simulink model "SrmUnlineSplineMat3"  (R2013b)
settings: Solver=ode45  StartTime=0.0  StopTime=2  MaxStep=5e-5  RelTol=1e-3
libraries: powerlib x26
settings Model: Creator=Administrator  LastModifiedBy=Think79
settings DataIOCC: SignalLoggingSaveFormat=ModelDataLogs
settings OptimizationCC: ExpressionDepthLimit=2147483647
settings DebuggingCC: FcnCallInpInsideContextMsg=UseLocalSettings  StateNameClashWarn=warning
settings GRTTargetCC: CombineOutputUpdateFcns=off  GRTInterface=on

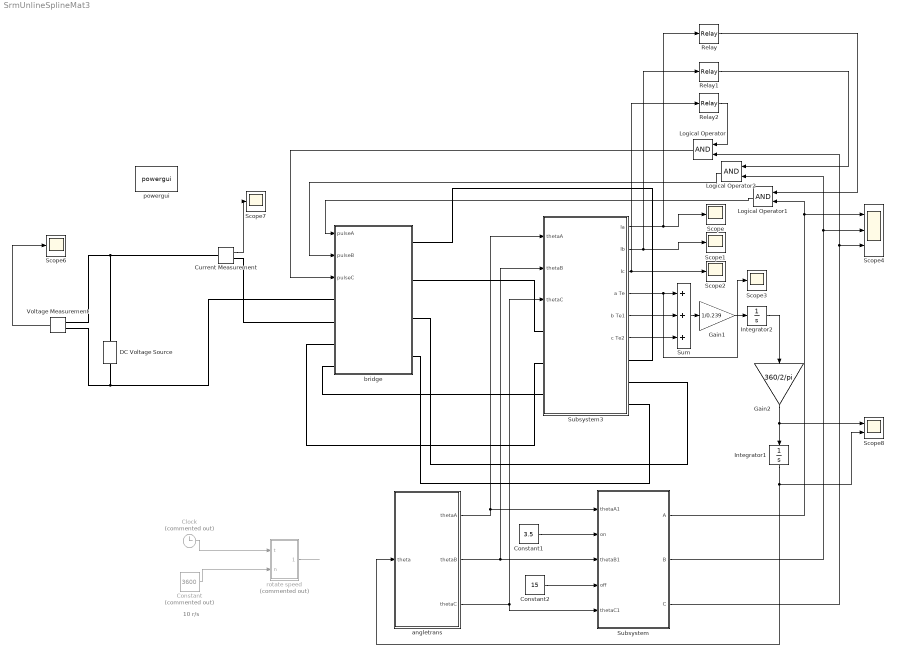
== system SrmUnlineSplineMat3 ==
  note: 10 r/s
  Clock : Clock  Commented=on
  Constant : Constant  Commented=on  Value=3600
  Constant1 : Constant  Value=3.5
  Constant2 : Constant  Value=15
  Current Measurement : powerlib/Measurements/Current Measurement  PhasorSimulation=off  OutputType=Complex  PSBequivalent=0
  DC Voltage Source : powerlib/Electrical Sources/DC Voltage Source  Amplitude=450  Measurements=None
  Gain1 : Gain  Gain=1/0.239
  Gain2 : Gain  Gain=360/2/pi
  Integrator1 : Integrator  InitialCondition=3.5
  Integrator2 : Integrator
  Logical Operator : Logic  AllPortsSameDT=off  OutDataTypeStr=boolean
  Logical Operator1 : Logic  AllPortsSameDT=off  OutDataTypeStr=boolean
  Logical Operator2 : Logic  AllPortsSameDT=off  OutDataTypeStr=boolean
  Relay : Relay  OnSwitchValue=32  OffSwitchValue=28  OnOutputValue=0  OffOutputValue=1
  Relay1 : Relay  OnSwitchValue=32  OffSwitchValue=28  OnOutputValue=0  OffOutputValue=1
  Relay2 : Relay  OnSwitchValue=32  OffSwitchValue=28  OnOutputValue=0  OffOutputValue=1
  Scope{,1..3,6..7} (6 alike) : Scope
      Scope settings: YMin=26  YMax=34
      Scope1 settings: YMin=0.00225  YMax=0.00225011
      Scope2 settings: YMin=0  YMax=1.75  SaveName=ScopeData2
      Scope3 settings: YMin=27  YMax=36  SaveName=ScopeData3
      Scope6 settings: YMin=39  YMax=41.5  SaveName=ScopeData8
      Scope7 settings: YMin=-1.75  YMax=2  SaveName=ScopeData12
  Scope4 : Scope  NumInputPorts=3
      settings: TimeRange=0.0001268631901574406  YMin=0~-1~-1  YMax=2~1~1  SaveName=ScopeData5
  Scope8 : Scope  NumInputPorts=2
      settings: YMin=2250~154  YMax=2340~164  SaveName=ScopeData16
  Subsystem : Subsystem
  Subsystem3 : Subsystem
  Sum : Sum  Inputs=+++
  Voltage Measurement : powerlib/Measurements/Voltage Measurement  PhasorSimulation=off  OutputType=Complex  PSBequivalent=0
  angletrans : Subsystem
  bridge : Subsystem
  powergui : powerlib/powergui  Priority=1  SimulationMode=Discrete  SolverType=Tustin  SampleTime=50e-6  frequency=60  SPID=off  DisableSnubberDevices=off  DisableRonSwitches=off  DisableVfSwitches=off  SwTol=0  Interpol=off  DisplayEquations=off  frequencyindice=0  Pbase=100e6  ErrMax=1e-4  Iterations=50  UnitsV=kV  UnitsW=MW  FunctionMessages=off  echomessages=off  HookPort=off  EnableUseOfTLC=off  x0status=blocks  RestoreLinks=warning  ResistiveCurrentMeasurement=off  Frange=[0:2:500]  Ylog=off  Xlog=on  ShowGrid=off  save=off  variable=ZData  ZoomFFT=on  StartTime=0.0  cycles=1  DisplayStyle=1  fundamental=60  FreqAxis=off  MaxFrequency=1000  frequencyindicesteady=1  RmsSteady=1  display=off  Ts=0  methode=off
  rotate speed : Subsystem  Commented=on
  wires:
  rotate speed/1(theta) -> ?
  Clock/1 -> rotate speed/1(t)
  Constant/1 -> rotate speed/2(n)
  Constant1/1 -> Subsystem/2(on)
  Constant2/1 -> Subsystem/4(off)
  angletrans/1(thetaA) -> Subsystem/1(thetaA1), Subsystem3/1(thetaA)
  angletrans/2(thetaB) -> Subsystem3/2(thetaB), Subsystem/3(thetaB1)
  angletrans/3(thetaC) -> Subsystem/5(thetaC1), Subsystem3/3(thetaC)
  Subsystem/1(A) -> Logical Operator1/2, Scope4/1
  Subsystem/3(C) -> Logical Operator/2, Scope4/3
  Subsystem3/1(Ia) -> Relay/1, Scope/1
  Subsystem3/3(Ic) -> Relay2/1, Scope2/1
  Subsystem3/2(Ib) -> Relay1/1, Scope1/1
  Voltage Measurement/1 -> Scope6/1
  Current Measurement/1 -> Scope7/1
  Subsystem3/4(a Te) -> Scope3/1, Sum/1
  Subsystem3/5(b Te1) -> Sum/2
  Subsystem3/6(c Te2) -> Sum/3
  Subsystem/2(B) -> Logical Operator2/2, Scope4/2
  Sum/1 -> Gain1/1
  Gain1/1 -> Integrator2/1
  Integrator1/1 -> Scope8/2, angletrans/1(theta)
  Integrator2/1 -> Gain2/1
  Gain2/1 -> Scope8/1, Integrator1/1
  Relay2/1 -> Logical Operator/1
  Logical Operator/1 -> bridge/3(pulseC)
  Relay1/1 -> Logical Operator2/1
  Logical Operator2/1 -> bridge/2(pulseB)
  Relay/1 -> Logical Operator1/1
  Logical Operator1/1 -> bridge/1(pulseA)
  connections:
  Current Measurement/LConn1 -- DC Voltage Source/RConn1 -- Voltage Measurement/LConn1
  bridge/LConn1 -- DC Voltage Source/LConn1 -- Voltage Measurement/LConn2
  bridge/RConn2 -- Subsystem3/LConn1
  bridge/RConn1 -- Subsystem3/RConn1
  bridge/LConn3 -- Subsystem3/LConn2
  bridge/LConn4 -- Subsystem3/LConn3
  bridge/RConn4 -- Subsystem3/RConn3
  bridge/RConn3 -- Subsystem3/RConn2
  Current Measurement/RConn1 -- bridge/LConn2

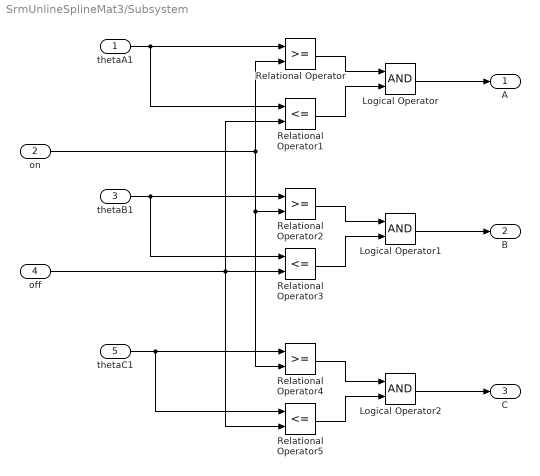
== system SrmUnlineSplineMat3/Subsystem ==
  thetaA1 : Inport
  on : Inport  Port=2
  thetaB1 : Inport  Port=3
  off : Inport  Port=4
  thetaC1 : Inport  Port=5
  Logical Operator : Logic  AllPortsSameDT=off  OutDataTypeStr=boolean
  Logical Operator1 : Logic  AllPortsSameDT=off  OutDataTypeStr=boolean
  Logical Operator2 : Logic  AllPortsSameDT=off  OutDataTypeStr=boolean
  Relational Operator : RelationalOperator  OutDataTypeStr=boolean
  Relational Operator1 : RelationalOperator  Operator=<=  OutDataTypeStr=boolean
  Relational Operator2 : RelationalOperator  OutDataTypeStr=boolean
  Relational Operator3 : RelationalOperator  Operator=<=  OutDataTypeStr=boolean
  Relational Operator4 : RelationalOperator  OutDataTypeStr=boolean
  Relational Operator5 : RelationalOperator  Operator=<=  OutDataTypeStr=boolean
  A : Outport
  B : Outport  Port=2
  C : Outport  Port=3
  wires:
  thetaA1/1 -> Relational Operator/1, Relational Operator1/1
  thetaB1/1 -> Relational Operator2/1, Relational Operator3/1
  thetaC1/1 -> Relational Operator4/1, Relational Operator5/1
  on/1 -> Relational Operator/2, Relational Operator2/2, Relational Operator4/2
  off/1 -> Relational Operator1/2, Relational Operator3/2, Relational Operator5/2
  Relational Operator/1 -> Logical Operator/1
  Relational Operator1/1 -> Logical Operator/2
  Relational Operator2/1 -> Logical Operator1/1
  Relational Operator3/1 -> Logical Operator1/2
  Relational Operator4/1 -> Logical Operator2/1
  Relational Operator5/1 -> Logical Operator2/2
  Logical Operator/1 -> A/1
  Logical Operator1/1 -> B/1
  Logical Operator2/1 -> C/1

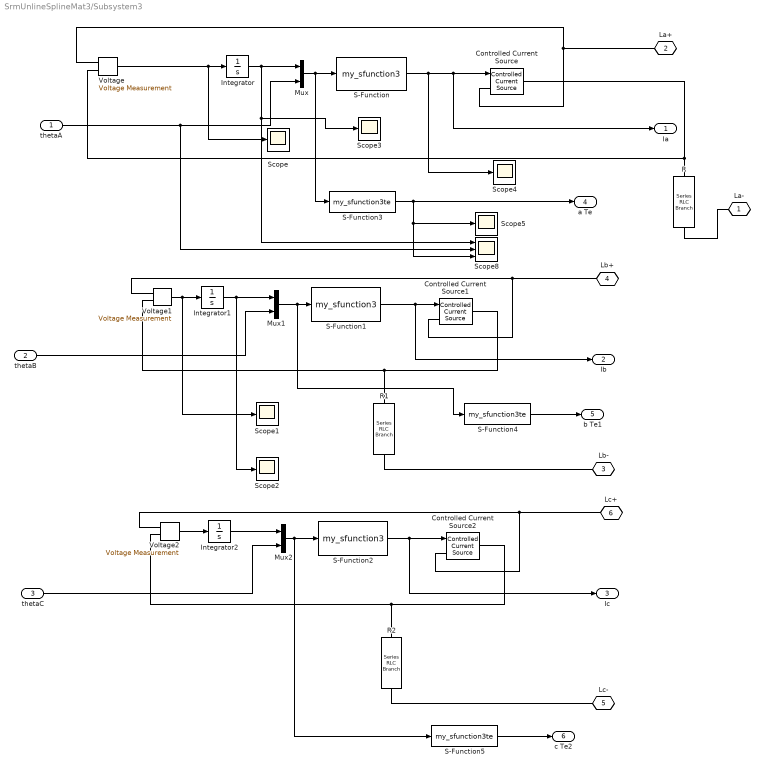
== system SrmUnlineSplineMat3/Subsystem3 ==
  thetaA : Inport
  thetaB : Inport  Port=2
  thetaC : Inport  Port=3
  Controlled Current Source : powerlib/Electrical Sources/Controlled Current Source  Initialize=on  Source_Type=AC  Amplitude=0  Phase=0  Frequency=0  Measurements=None
  Controlled Current Source1 : powerlib/Electrical Sources/Controlled Current Source  Initialize=on  Source_Type=AC  Amplitude=0  Phase=0  Frequency=0  Measurements=None
  Controlled Current Source2 : powerlib/Electrical Sources/Controlled Current Source  Initialize=on  Source_Type=AC  Amplitude=0  Phase=0  Frequency=0  Measurements=None
  Integrator : Integrator  LimitOutput=on  LowerSaturationLimit=0
  Integrator1 : Integrator  LimitOutput=on  LowerSaturationLimit=0
  Integrator2 : Integrator  LimitOutput=on  LowerSaturationLimit=0
  Mux : Mux  Inputs=2
  Mux1 : Mux  Inputs=2
  Mux2 : Mux  Inputs=2
  R : powerlib/Elements/Series RLC Branch  LConnTagsString=__new0  RConnTagsString=__new0  BranchType=R  Resistance=0.0261014  Inductance=1.0  SetiL0=off  InitialCurrent=0  Capacitance=1.0  Setx0=off  InitialVoltage=0  Measurements=None
  R1 : powerlib/Elements/Series RLC Branch  LConnTagsString=__new0  RConnTagsString=__new0  BranchType=R  Resistance=0.0261014  Inductance=1.0  SetiL0=off  InitialCurrent=0  Capacitance=1.0  Setx0=off  InitialVoltage=0  Measurements=None
  R2 : powerlib/Elements/Series RLC Branch  LConnTagsString=__new0  RConnTagsString=__new0  BranchType=R  Resistance=0.0261014  Inductance=1.0  SetiL0=off  InitialCurrent=0  Capacitance=1.0  Setx0=off  InitialVoltage=0  Measurements=None
  S-Function : S-Function  FunctionName=my_sfunction3  EnableBusSupport=off
  S-Function1 : S-Function  FunctionName=my_sfunction3  EnableBusSupport=off
  S-Function2 : S-Function  FunctionName=my_sfunction3  EnableBusSupport=off
  S-Function3 : S-Function  FunctionName=my_sfunction3te  EnableBusSupport=off
  S-Function4 : S-Function  FunctionName=my_sfunction3te  EnableBusSupport=off
  S-Function5 : S-Function  FunctionName=my_sfunction3te  EnableBusSupport=off
  Scope{,1..5} (6 alike) : Scope
      Scope settings: YMin=-500  YMax=500  SaveName=ScopeData4
      Scope1 settings: YMin=-2.25  YMax=0.75  SaveName=ScopeData9
      Scope2 settings: YMin=-2.25  YMax=0.75  SaveName=ScopeData10
      Scope3 settings: YMin=-2.25  YMax=0.75  SaveName=ScopeData11
      Scope4 settings: YMin=0  YMax=13  SaveName=ScopeData13
      Scope5 settings: YMin=-3.4e-07  YMax=-2.85e-07  SaveName=ScopeData14
  Scope8 : Scope  NumInputPorts=3
      settings: YMin=0~0~-200  YMax=2~45~500  SaveName=ScopeData15
  Voltage : powerlib/Measurements/Voltage Measurement  PhasorSimulation=off  OutputType=Complex  PSBequivalent=0
  Voltage1 : powerlib/Measurements/Voltage Measurement  PhasorSimulation=off  OutputType=Complex  PSBequivalent=0
  Voltage2 : powerlib/Measurements/Voltage Measurement  PhasorSimulation=off  OutputType=Complex  PSBequivalent=0
  La- : PMIOPort  Tag=PMCPort  Port=1  Side=Left
  La+ : PMIOPort  Tag=PMCPort  Port=2  Side=Right
  Lb- : PMIOPort  Tag=PMCPort  Port=3  Side=Left
  Lb+ : PMIOPort  Tag=PMCPort  Port=4  Side=Right
  Lc- : PMIOPort  Tag=PMCPort  Port=5  Side=Left
  Lc+ : PMIOPort  Tag=PMCPort  Port=6  Side=Right
  Ia : Outport
  Ib : Outport  Port=2
  Ic : Outport  Port=3
  a Te : Outport  Port=4
  b Te1 : Outport  Port=5
  c Te2 : Outport  Port=6
  wires:
  Mux/1 -> S-Function3/1, S-Function/1
  Integrator/1 -> Mux/1, Scope8/1, Scope3/1
  thetaA/1 -> Scope8/2, Mux/2
  Voltage/1 -> Integrator/1, Scope/1
  Mux1/1 -> S-Function4/1, S-Function1/1
  Integrator1/1 -> Mux1/1, Scope2/1
  thetaB/1 -> Mux1/2
  S-Function1/1 -> Controlled Current Source1/1, Ib/1
  Voltage1/1 -> Integrator1/1, Scope1/1
  Mux2/1 -> S-Function5/1, S-Function2/1
  Integrator2/1 -> Mux2/1
  thetaC/1 -> Mux2/2
  S-Function2/1 -> Controlled Current Source2/1, Ic/1
  Voltage2/1 -> Integrator2/1
  S-Function/1 -> Scope4/1, Ia/1, Controlled Current Source/1
  S-Function3/1 -> Scope8/3, Scope5/1, a Te/1
  S-Function4/1 -> b Te1/1
  S-Function5/1 -> c Te2/1
  connections:
  Controlled Current Source/LConn1 -- Voltage/LConn1 -- La+/RConn1
  La-/RConn1 -- R/RConn1
  Lb+/RConn1 -- Voltage1/LConn1 -- Controlled Current Source1/LConn1
  Lb-/RConn1 -- R1/RConn1
  Controlled Current Source1/RConn1 -- R1/LConn1 -- Voltage1/LConn2
  Lc+/RConn1 -- Voltage2/LConn1 -- Controlled Current Source2/LConn1
  Lc-/RConn1 -- R2/RConn1
  Controlled Current Source2/RConn1 -- R2/LConn1 -- Voltage2/LConn2
  Controlled Current Source/RConn1 -- Voltage/LConn2 -- R/LConn1

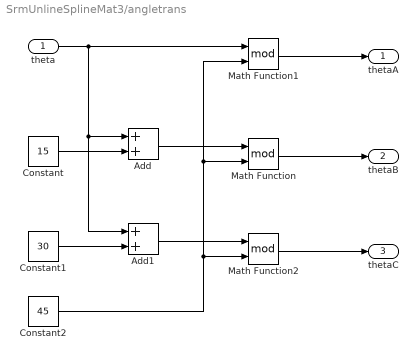
== system SrmUnlineSplineMat3/angletrans ==
  theta : Inport
  Add : Sum
  Add1 : Sum
  Constant : Constant  Value=15
  Constant1 : Constant  Value=30
  Constant2 : Constant  Value=45
  Math Function : Math  Operator=mod  SaturateOnIntegerOverflow=on
  Math Function1 : Math  Operator=mod  SaturateOnIntegerOverflow=on
  Math Function2 : Math  Operator=mod  SaturateOnIntegerOverflow=on
  thetaA : Outport
  thetaB : Outport  Port=2
  thetaC : Outport  Port=3
  wires:
  Add1/1 -> Math Function2/1
  Add/1 -> Math Function/1
  theta/1 -> Math Function1/1, Add1/1, Add/1
  Constant/1 -> Add/2
  Constant1/1 -> Add1/2
  Constant2/1 -> Math Function2/2, Math Function/2, Math Function1/2
  Math Function2/1 -> thetaC/1
  Math Function/1 -> thetaB/1
  Math Function1/1 -> thetaA/1

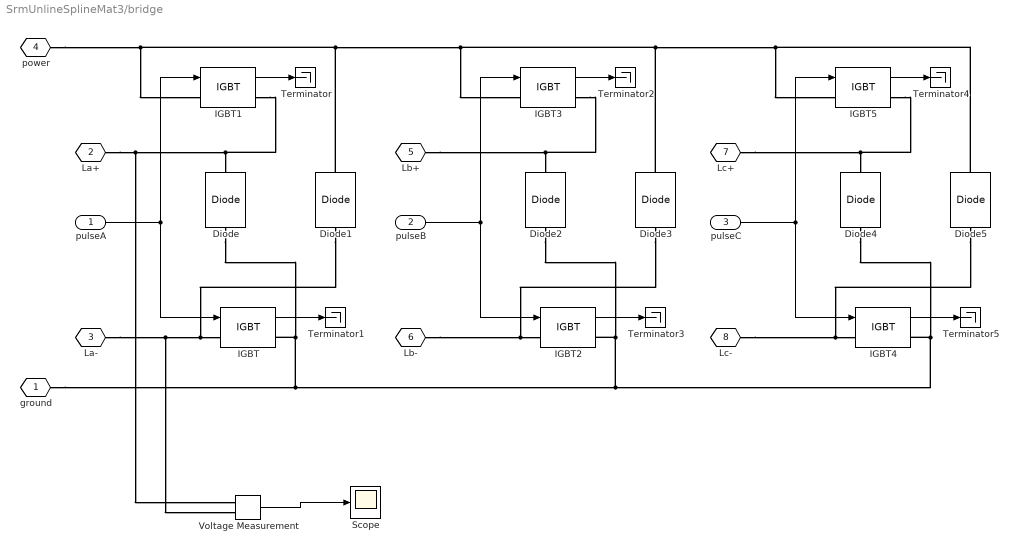
== system SrmUnlineSplineMat3/bridge ==
  pulseA : Inport
  pulseB : Inport  Port=2
  pulseC : Inport  Port=3
  Diode{,1..5} (6 alike) : powerlib/Power Electronics/Diode  Ron=0.001  Lon=0  Vf=0.8  IC=0  UseSnubber=off  Rs=500  Cs=250e-9  Measurements=off
  IGBT{,1..5} (6 alike) : powerlib/Power Electronics/IGBT  Ron=0.001  Lon=0  Vf=1  Tf=1e-6  Tt=2e-6  IC=0  Rs=1e5  Cs=inf  Measurements=on
  Scope : Scope
      settings: YMin=57.14  YMax=57.2  SaveName=ScopeData6
  Terminator{,1..5} (6 alike) : Terminator
  Voltage Measurement : powerlib/Measurements/Voltage Measurement  PhasorSimulation=off  OutputType=Complex  PSBequivalent=0
  ground : PMIOPort  Tag=PMCPort  Port=1  Side=Left
  La+ : PMIOPort  Tag=PMCPort  Port=2  Side=Right
  La- : PMIOPort  Tag=PMCPort  Port=3  Side=Right
  power : PMIOPort  Tag=PMCPort  Port=4  Side=Left
  Lb+ : PMIOPort  Tag=PMCPort  Port=5  Side=Right
  Lb- : PMIOPort  Tag=PMCPort  Port=6  Side=Left
  Lc+ : PMIOPort  Tag=PMCPort  Port=7  Side=Right
  Lc- : PMIOPort  Tag=PMCPort  Port=8  Side=Left
  wires:
  IGBT4/1 -> Terminator5/1
  IGBT5/1 -> Terminator4/1
  pulseC/1 -> IGBT4/1, IGBT5/1
  IGBT2/1 -> Terminator3/1
  IGBT3/1 -> Terminator2/1
  pulseB/1 -> IGBT2/1, IGBT3/1
  IGBT/1 -> Terminator1/1
  IGBT1/1 -> Terminator/1
  pulseA/1 -> IGBT/1, IGBT1/1
  Voltage Measurement/1 -> Scope/1
  connections:
  Lc-/RConn1 -- Diode5/LConn1 -- IGBT4/LConn1
  Lc+/RConn1 -- IGBT5/RConn1 -- Diode4/RConn1
  Lb-/RConn1 -- Diode3/LConn1 -- IGBT2/LConn1
  Lb+/RConn1 -- IGBT3/RConn1 -- Diode2/RConn1
  Diode5/RConn1 -- IGBT5/LConn1 -- Diode3/RConn1 -- IGBT3/LConn1 -- Diode1/RConn1 -- IGBT1/LConn1 -- power/RConn1
  La-/RConn1 -- Diode1/LConn1 -- IGBT/LConn1 -- Voltage Measurement/LConn2
  La+/RConn1 -- IGBT1/RConn1 -- Diode/RConn1 -- Voltage Measurement/LConn1
  IGBT2/RConn1 -- Diode2/LConn1 -- IGBT/RConn1 -- Diode/LConn1 -- ground/RConn1 -- IGBT4/RConn1 -- Diode4/LConn1

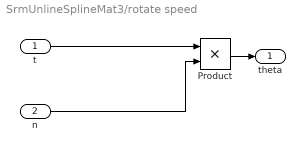
== system SrmUnlineSplineMat3/rotate speed ==
  t : Inport
  n : Inport  Port=2
  Product : Product  RndMeth=Zero
  theta : Outport
  wires:
  n/1 -> Product/2
  t/1 -> Product/1
  Product/1 -> theta/1
